simulink model "pressure_regulator_step_response"  (R2019b)
settings: Solver=ode3  StartTime=0.0  StopTime=0.5  FixedStep=1e-5  RelTol=1e-3
settings Model: Creator=Alexander  LastModifiedBy=Alexander
settings SolverCC: InsertRTBMode=Never (minimum delay)
settings DataIOCC: SaveFormat=Array  SaveTime=off  OutputSaveName=reduced_pressure
settings RTWCC: PackageGeneratedCodeAndArtifacts=on  BuildConfiguration=Faster Runs

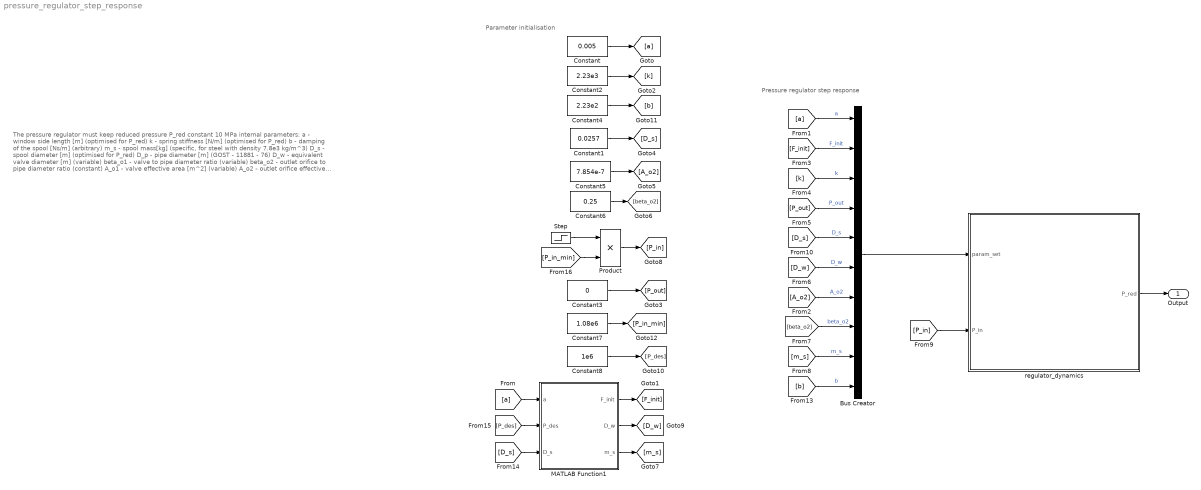
== system pressure_regulator_step_response ==
  note: Pressure regulator step response
  note: The pressure regulator must keep reduced pressure P_red constant 10 MPa
      |
      | internal parameters:
      | a - window side length [m] (optimised for P_red)
      | k - spring stiffness [N/m] (optimised for P_red)
      | b - damping of the spool [Ns/m] (arbitrary)
      | m_s - spool mass[kg] (specific, for steel with density 7.8e3 kg/m^3)
      |
      | D_s - spool diameter [m] (optimised for P_red)
      | D_p - pipe diameter [m] (GOST - 11881 - 76)
      | D_w - equivalent valve diameter [m] (variable)
      |
      | beta_o1 - valve to pipe diameter ratio (variable)
      | beta_o2 - outlet orifice to pipe diameter ratio (constant)
      |
      | A_o1 - valve effective area [m^2] (variable)
      | A_o2 - outlet orifice effective area [m^2] (constant)
      |
      | P_in - inlet pressure [Pa] (variable, gauge)
      | P_out - outlet pressure [Pa] (constant, ambient, gauge)
      | P_in_min - minimum operational pressure on the inlet [Pa] (specific, constant)
      | P_des - desired reduced pressure [Pa] (given)
      |
      | F_init - initial force on the spool [N] (constant)
  note: Parameter initialisation
  Bus Creator : BusCreator  Inputs=10
  Constant : Constant  Value=0.005
  Constant1 : Constant  Value=0.0257
  Constant2 : Constant  Value=2.23e3
  Constant3 : Constant  Value=0
  Constant4 : Constant  Value=2.23e2
  Constant5 : Constant  Value=7.854e-7
  Constant6 : Constant  Value=0.25
  Constant7 : Constant  Value=1.08e6
  Constant8 : Constant  Value=1e6
  MATLAB Function1 : MATLAB Function  TreatAsAtomicUnit=on
  Product : Product
  Step : Step  Time=0.1  Before=1  After=2  SampleTime=0
  regulator_dynamics : Subsystem
  Output : Outport  SignalName=P_red  OutDataTypeStr=double
  wires:
  Constant8/1 -> [P_des]
  Constant1/1 -> [D_s]
  Constant6/1 -> [beta_o2]
  Product/1 -> [P_in]
  [a] -> Bus Creator/1  "a"
  [P_out] -> Bus Creator/4  "P_out"
  [P_in_min] -> Product/2
  [D_s] -> Bus Creator/5  "D_s"
  [a] -> MATLAB Function1/1(a)
  Constant7/1 -> [P_in_min]
  Step/1 -> Product/1
  [D_w] -> Bus Creator/6  "D_w"
  [P_in] -> regulator_dynamics/2(P_in)
  [A_o2] -> Bus Creator/7  "A_o2"
  MATLAB Function1/2(D_w) -> [D_w]
  Constant/1 -> [a]
  Constant5/1 -> [A_o2]
  [k] -> Bus Creator/3  "k"
  [F_init] -> Bus Creator/2  "F_init"
  Constant4/1 -> [b]
  MATLAB Function1/3(m_s) -> [m_s]
  [b] -> Bus Creator/10  "b"
  Bus Creator/1 -> regulator_dynamics/1(param_set)
  [beta_o2] -> Bus Creator/8  "beta_o2"
  Constant3/1 -> [P_out]
  [D_s] -> MATLAB Function1/3(D_s)
  [P_des] -> MATLAB Function1/2(P_des)
  Constant2/1 -> [k]
  [m_s] -> Bus Creator/9  "m_s"
  regulator_dynamics/1(P_red) -> Output/1
  MATLAB Function1/1(F_init) -> [F_init]

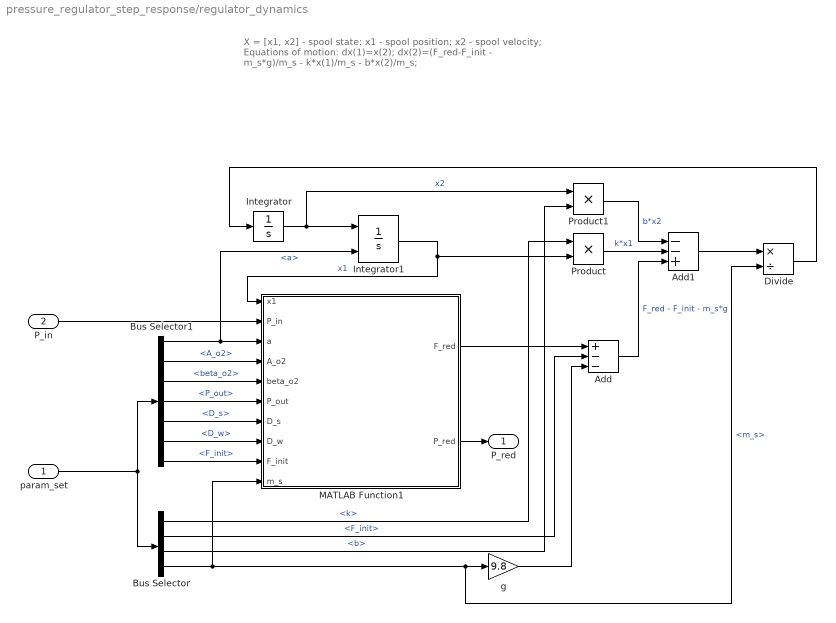
== system pressure_regulator_step_response/regulator_dynamics ==
  note: X = [x1, x2] - spool state:
      | 	x1 - spool position;
      | 	x2 - spool velocity;
      |
      | Equations of motion:
      | dx(1)=x(2);
      | dx(2)=(F_red-F_init - m_s*g)/m_s - k*x(1)/m_s - b*x(2)/m_s;
  param_set : Inport
  P_in : Inport  Port=2
  Add : Sum  Inputs=+--
  Add1 : Sum  Inputs=--+
  Bus Selector : BusSelector  OutputSignals=k,F_init,b,m_s
  Bus Selector1 : BusSelector  OutputSignals=a,A_o2,beta_o2,P_out,D_s,D_w,F_init
  Divide : Product  Inputs=*/
  Integrator : Integrator
  Integrator1 : Integrator  InitialConditionSource=external
  MATLAB Function1 : MATLAB Function  TreatAsAtomicUnit=on
  Product : Product
  Product1 : Product
  g : Gain  Gain=9.8
  P_red : Outport
  wires:
  MATLAB Function1/2(P_red) -> P_red/1
  P_in/1 -> MATLAB Function1/2(P_in)
  Add/1 -> Add1/3  "F_red - F_init - m_s*g"
  MATLAB Function1/1(F_red) -> Add/1
  Integrator/1 -> Product1/1, Integrator1/1  "x2"
  Product/1 -> Add1/2  "k*x1"
  Divide/1 -> Integrator/1
  Add1/1 -> Divide/1
  param_set/1 -> Bus Selector/1, Bus Selector1/1
  Bus Selector/1 -> Product/1  "<k>"
  Bus Selector/2 -> Add/2  "<F_init>"
  Integrator1/1 -> MATLAB Function1/1(x1), Product/2  "x1"
  Bus Selector1/7 -> MATLAB Function1/9(F_init)  "<F_init>"
  Bus Selector1/6 -> MATLAB Function1/8(D_w)  "<D_w>"
  Bus Selector1/5 -> MATLAB Function1/7(D_s)  "<D_s>"
  Bus Selector1/4 -> MATLAB Function1/6(P_out)  "<P_out>"
  Bus Selector1/3 -> MATLAB Function1/5(beta_o2)  "<beta_o2>"
  Bus Selector1/2 -> MATLAB Function1/4(A_o2)  "<A_o2>"
  Bus Selector1/1 -> Integrator1/2, MATLAB Function1/3(a)  "<a>"
  Bus Selector/3 -> Product1/2  "<b>"
  Product1/1 -> Add1/1  "b*x2"
  Bus Selector/4 -> MATLAB Function1/10(m_s), Divide/2, g/1  "<m_s>"
  g/1 -> Add/3

== matlab function pressure_regulator_step_response/regulator_dynamics/MATLAB Function1 ==
  data: x1 input; F_red output; P_in input; a input; A_o2 input; P_red output; beta_o2 input; P_out input; D_s input; D_w input; F_init input; m_s input
function [F_red, P_red]  = reduced_pressure_force(x1, P_in, a, ...
                            A_o2, beta_o2, P_out, D_s, D_w, F_init, m_s)
% current reduced pressure force calculation
%%

% calculate effective valve area
alpha = 2*asin(a/D_s);              % angular extent of the window
l = (D_s/2)*alpha;                  % circumferential length of the window
A_o1 = l*(a-x1);                    % current area of the valve

if A_o1<0, A_o1 = 0;
end                                 % valve closes if x(1)>a, so A_o1 is non-negative

beta_o1 = sqrt(4*A_o1/pi)/D_w;      % current area of the valve/pipe

gamma_1 = A_o1^2*(1-beta_o2^4);
gamma_2 = A_o2^2*(1-beta_o1^4);
% calculate current reduced pressure
P_red = (gamma_1*P_in + gamma_2*P_out)/(gamma_1 + gamma_2);
% and reduced pressure force on the spool, assuming it acts on the whole
% surface, i.e. shoulder area is neglected (unlike the shoulder force)

F_red = P_red*(pi*D_s^2)/4;

if F_red<(F_init+m_s*9.8)
    F_red = F_init+m_s*9.8;
end
end

== matlab function pressure_regulator_step_response/MATLAB Function1 ==
  data: F_init output; a input; P_des input; D_w output; m_s output; D_s input
function [F_init, D_w, m_s] = param_init(a, P_des, D_s)
% function initializes all parameters that depend on the variable
% parameters of the window size 'a' 
%%
F_init = 0.98*P_des*(pi*D_s^2)/4;              % initial force on the spool
D_w = sqrt(4*a^2/pi);                   % equivalent diameter of the window

% calculate spool volume
V_s = 2*a*(pi*(3*a)^2)/4 + 3*a*(pi*(1.5*a)^2)/4;

% calculate spool mass
rho = 7.8e3;
m_s = V_s*rho;
